simulink model "E_hyeok_RateError"  (R2023b)
settings: Solver=FixedStepAuto  StartTime=0.0  StopTime=inf  FixedStep=0.001  RelTol=1e-3  EnableMultiTasking=on
libraries: arduinolib x12, simulink x3, dspswit3 x2, spsOnDelayLib x2, arduinosensorlib x1
settings Model: ExtModeTrigDuration=2  Creator=user  LastModifiedBy=현대오토1
settings OptimizationCC: EnhancedBackFolding=on  PassReuseOutputArgsAs=Individual arguments  ZeroExternalMemoryAtStartup=off  ZeroInternalMemoryAtStartup=off  MaxStackSize=64  OptimizeBlockOrder=speed  DifferentSizesBufferReuse=on  OptimizationCustomize=off  EfficientTunableParamExpr=on
settings DebuggingCC: ParameterTunabilityLossMsg=error
settings HardwareCC: ProdBitPerInt=16  ProdBitPerPointer=16  ProdBitPerSizeT=16  ProdBitPerPtrDiffT=16  ProdLargestAtomicFloat=None  ProdWordSize=8  ProdHWDeviceType=Atmel->AVR
settings SFSimCC: MATLABDynamicMemAlloc=off
settings RTWCC: Description=Embedded Coder  SystemTargetFile=ert.tlc  HardwareBoard=Arduino Mega 2560  TemplateMakefile=ert_default_tmf  Toolchain=Arduino AVR  BuildConfiguration=Faster Runs
settings CodeAppCC: ForceParamTrailComments=on  IgnoreCustomStorageClasses=off  OperatorAnnotations=on  SimulinkDataObjDesc=on  SFDataObjDesc=on  InsertBlockDesc=on
settings ERTTargetCC: SupportContinuousTime=on  SupportVariableSizeSignals=on  ExtModeTransport=3  ExtModeStaticAlloc=on  ExtModeAutomaticAllocSize=off  ExtModeStaticAllocSize=2048  ExtModeMexFile=ext_xcp  ExtModeIntrfLevel=Level2 - Open

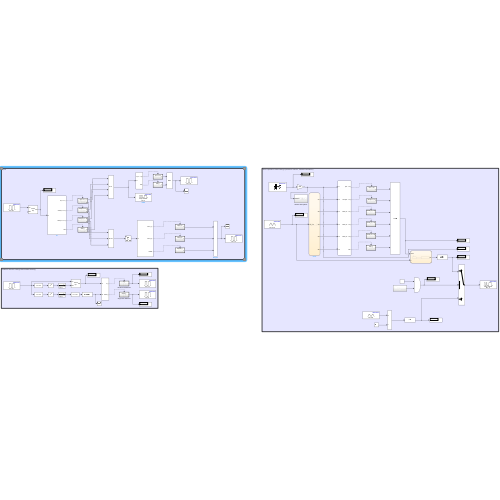
[thumbnail: Simulink's stored preview of the top-level diagram]
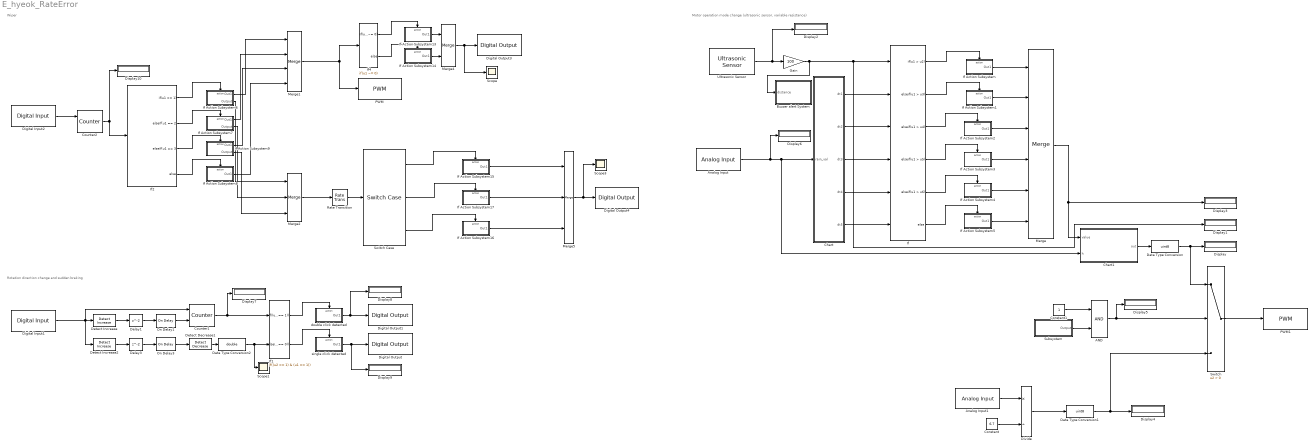
== system E_hyeok_RateError ==
  note: Wiper
  note: Motor operation mode change (ultrasonic sensor, variable resistance)
  note: Rotation direction change and sudden braking
  AND : Logic  IconShape=distinctive  AllPortsSameDT=off  OutDataTypeStr=boolean
  Analog Input : arduinolib/Analog Input  pinNumber=10  ReadResultsOnly=off  ConversionTriggerSource=Software  ExternalTriggerType=uint32( 0 )  OutputDataType=uint16  EnableConversionCompleteNotify=off  EnableOuputStatus=off  SampleTime=-1  blockPlatform=arduino
  Analog Input1 : arduinolib/Analog Input  pinNumber=8  ReadResultsOnly=off  ConversionTriggerSource=Software  ExternalTriggerType=uint32( 0 )  OutputDataType=uint16  EnableConversionCompleteNotify=off  EnableOuputStatus=off  SampleTime=-1  blockPlatform=arduino
  Buzzer alert System : Subsystem
  Chart : Stateflow chart  TreatAsAtomicUnit=on
  Chart1 : Stateflow chart  TreatAsAtomicUnit=on
      settings: PortSchema="{\"entries\":[{\"content\":{\"sides\":[{\"content\":{\"connectorIds\":[\"In2\",\"In1\"]},\"type\":\"ConnectorPlacement.EquallySpacedRectSide\",\"uuid\":\"b8bc21d1-4b9f-4189-a812-b41a4c5af9e6\"},{\"content\":{\"connectorIds\":[\"Out1\"],\"side\":\"RIGHT\"},\"type\":\"ConnectorPlacement.EquallySpacedRectSide\",\"uuid\":\"2c64dce3-08c2-4220-8c60-db9aba55cb61\"},{\"content\":{\"connectorIds\":[],\"side\":\"TOP\"},\"type\":\"ConnectorPlacement.EquallySpacedRectSide\",\"uuid\":\"e1e14768-a3b4-4969-ba09-2d2b4c878f0a\"}]},\"type\":\"ConnectorPlacement.EquallySpacedConnector\",\"uuid\":\"33700ad2-0727-43da-b85e-9713a6dc3065\"}],\"packageUris\":[\"http://schema.mathworks.com/mf0/Connector/R2020b\"],\"version\":\"1.0\"}"
  Constant : Constant  Value=6.7
  Constant1 : Constant
  Counter1 : dspswit3/Counter  Direction=Up  CountEvent=Rising edge  CounterSize=User defined  MaxCount=255  InitialCount=0  Output=Count  HitValue=32  ResetInput=on  SamplesPerFrame=1  Ts=1  CntDtype=double  HitDtype=Logical
  Counter2 : dspswit3/Counter  Direction=Up  CountEvent=Falling edge  CounterSize=User defined  MaxCount=3  InitialCount=0  Output=Count  HitValue=32  ResetInput=on  SamplesPerFrame=1  Ts=1  CntDtype=int8  HitDtype=Logical
  Data Type Conversion : DataTypeConversion  OutDataTypeStr=uint8  SaturateOnIntegerOverflow=off  RndMeth=Floor
  Data Type Conversion1 : DataTypeConversion  OutDataTypeStr=uint8  SaturateOnIntegerOverflow=off  RndMeth=Floor
  Data Type Conversion2 : DataTypeConversion  OutDataTypeStr=double  SaturateOnIntegerOverflow=off  RndMeth=Floor
  Delay1 : Delay
  Delay3 : Delay
  Detect Decrease1 : simulink/Logic and Bit Operations/Detect Decrease  vinit=0  OutDataTypeStr=uint8
  Detect Increase : simulink/Logic and Bit Operations/Detect Increase  vinit=1  OutDataTypeStr=boolean
  Detect Increase2 : simulink/Logic and Bit Operations/Detect Increase  vinit=1  OutDataTypeStr=boolean
  Digital Input1 : arduinolib/Digital Input  pinNumber=22  mode=Default  Direction=input  SampleTime=0.001  blockPlatform=arduino
  Digital Input2 : arduinolib/Digital Input  pinNumber=36  mode=Default  Direction=input  SampleTime=0.01  blockPlatform=arduino
  Digital Output : arduinolib/Digital Output  pinNumber=8  Direction=output  blockPlatform=arduino
  Digital Output1 : arduinolib/Digital Output  pinNumber=13  Direction=output  blockPlatform=arduino
  Digital Output3 : arduinolib/Digital Output  pinNumber=18  Direction=output  blockPlatform=arduino
  Digital Output4 : arduinolib/Digital Output  pinNumber=12  Direction=output  blockPlatform=arduino
  Display{,1..10} (11 alike) : Display
  Divide : Product  Inputs=*/
  Gain : Gain  Gain=100
  If : If  NumInputs=6  IfExpression=u1 > u2  ElseIfExpressions=u1 > u3, u1 > u4, u1 > u5, u1 > u6
  If Action Subsystem : Subsystem  TreatAsAtomicUnit=on
  If Action Subsystem1 : Subsystem  TreatAsAtomicUnit=on
  If Action Subsystem13 : Subsystem  TreatAsAtomicUnit=on
  If Action Subsystem14 : Subsystem  TreatAsAtomicUnit=on
  If Action Subsystem15 : Subsystem  TreatAsAtomicUnit=on
  If Action Subsystem16 : Subsystem  TreatAsAtomicUnit=on
  If Action Subsystem17 : Subsystem  TreatAsAtomicUnit=on
  If Action Subsystem2 : Subsystem  TreatAsAtomicUnit=on
  If Action Subsystem3 : Subsystem  TreatAsAtomicUnit=on
  If Action Subsystem4 : Subsystem  TreatAsAtomicUnit=on
  If Action Subsystem5 : Subsystem  TreatAsAtomicUnit=on
  If Action Subsystem6 : Subsystem  TreatAsAtomicUnit=on
  If Action Subsystem7 : Subsystem  TreatAsAtomicUnit=on
  If Action Subsystem8 : Subsystem  TreatAsAtomicUnit=on
  If Action Subsystem9 : Subsystem  TreatAsAtomicUnit=on
  If1 : If  NumInputs=2  IfExpression=(u2 == 1) & (u1 == 1)  ElseIfExpressions=(u2 == 1) & (u1 == 0)  ShowElse=off
  If2 : If  IfExpression=u1 == 1  ElseIfExpressions=u1 == 2, u1 == 3
  If4 : If  IfExpression=u1 ~= 0
  Merge : Merge  Inputs=6
  Merge1 : Merge  Inputs=4
  Merge2 : Merge  Inputs=3
  Merge4 : Merge
  Merge5 : Merge  Inputs=3
  On Delay1 : spsOnDelayLib/On Delay  DelayType=Off delay  delay=0.9  ic=0  Ts=0
  On Delay3 : spsOnDelayLib/On Delay  DelayType=Off delay  delay=0.9  ic=0  Ts=0
  PWM : arduinolib/PWM  pinNumber=3  frequencyType=Default  desiredFrequency=490.2  achievableFrequency=490.2
  PWM1 : arduinolib/PWM  pinNumber=11  frequencyType=Default  desiredFrequency=490.2  achievableFrequency=490.2
  Rate Transition : RateTransition  InitialCondition=0.01  OutPortSampleTime=0.001
  Scope : Scope
  Scope1 : Scope
  Scope3 : Scope
  Subsystem : Subsystem
  Switch : Switch  Criteria=u2 > Threshold  SaturateOnIntegerOverflow=off  InputSameDT=off
  Switch Case : SwitchCase  CaseConditions={1, 2}
  Ultrasonic Sensor : arduinosensorlib/Ultrasonic Sensor  NumSignalPins=2  TrigPin=50  EchoPin=51  SignalPin=3  SampleTime_=0.1  blockPlatform=ARDUINO
  double click detected : Subsystem  TreatAsAtomicUnit=on
  single click detected : Subsystem  TreatAsAtomicUnit=on
  wires:
  Ultrasonic Sensor/1 -> Gain/1, Display2/1
  Chart/1(dt1) -> If/2
  Chart/2(dt2) -> If/3
  Chart/3(dt3) -> If/4
  Chart/5(dt5) -> If/6
  Chart/4(dt4) -> If/5
  If Action Subsystem/1(Out1) -> Merge/1
  Gain/1 -> Buzzer alert System/1(distance), Display1/1, If/1
  If/2 -> If Action Subsystem1/Action
  If/3 -> If Action Subsystem2/Action
  If/4 -> If Action Subsystem3/Action
  If/5 -> If Action Subsystem4/Action
  If/6 -> If Action Subsystem5/Action
  If/1 -> If Action Subsystem/Action
  If Action Subsystem1/1(Out1) -> Merge/2
  If Action Subsystem2/1(Out1) -> Merge/3
  If Action Subsystem3/1(Out1) -> Merge/4
  If Action Subsystem4/1(Out1) -> Merge/5
  If Action Subsystem5/1(Out1) -> Merge/6
  Merge/1 -> Chart1/2(value), Display3/1
  Analog Input/1 -> Display6/1, Chart1/1(h), Chart/1(rain_val)
  Chart1/1(out) -> Data Type Conversion/1
  Data Type Conversion/1 -> Switch/1, Display/1
  AND/1 -> Display5/1, Switch/2
  Divide/1 -> Data Type Conversion1/1
  Switch/1 -> PWM1/1
  Constant1/1 -> AND/1
  Data Type Conversion1/1 -> Switch/3, Display4/1
  Constant/1 -> Divide/2
  Subsystem/1(Output) -> AND/2
  Analog Input1/1 -> Divide/1
  Detect Decrease1/1 -> Data Type Conversion2/1
  On Delay3/1 -> Detect Decrease1/1
  single click detected/1(Out1) -> Digital Output/1, Display9/1
  Detect Increase2/1 -> Delay3/1
  Delay3/1 -> On Delay3/1
  If1/2 -> single click detected/Action
  If1/1 -> double click detected/Action
  Counter1/1 -> Display7/1, If1/1
  Delay1/1 -> On Delay1/1
  Detect Increase/1 -> Delay1/1
  Data Type Conversion2/1 -> Scope1/1, If1/2
  Digital Input1/1 -> Counter1/1, Detect Increase2/1, Detect Increase/1
  double click detected/1(Out1) -> Digital Output1/1, Display8/1
  On Delay1/1 -> Counter1/2
  Merge4/1 -> Scope/1, Digital Output3/1
  If Action Subsystem7/2(Output) -> Merge2/2
  If Action Subsystem6/2(Output) -> Merge2/1
  If Action Subsystem14/1(Out1) -> Merge4/2
  If Action Subsystem13/1(Out1) -> Merge4/1
  Counter2/1 -> Display10/1, If2/1
  Merge1/1 -> If4/1, PWM/1
  If Action Subsystem9/2(Output) -> Merge2/3
  If2/4 -> If Action Subsystem8/Action
  Digital Input2/1 -> Counter2/1
  If2/1 -> If Action Subsystem6/Action
  If2/2 -> If Action Subsystem7/Action
  If2/3 -> If Action Subsystem9/Action
  If Action Subsystem6/1(Out1) -> Merge1/1
  If Action Subsystem7/1(Out1) -> Merge1/2
  If Action Subsystem9/1(Out1) -> Merge1/3
  If Action Subsystem8/1(Out1) -> Merge1/4
  If4/2 -> If Action Subsystem14/Action
  If4/1 -> If Action Subsystem13/Action
  Merge2/1 -> Rate Transition/1
  Merge5/1 -> Scope3/1, Digital Output4/1
  If Action Subsystem16/1(Out1) -> Merge5/3
  If Action Subsystem17/1(Out1) -> Merge5/2
  If Action Subsystem15/1(Out1) -> Merge5/1
  Switch Case/1 -> If Action Subsystem15/Action
  Switch Case/2 -> If Action Subsystem17/Action
  Switch Case/3 -> If Action Subsystem16/Action
  Rate Transition/1 -> Switch Case/1

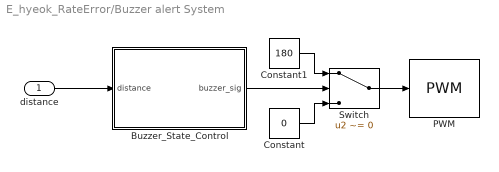
== system E_hyeok_RateError/Buzzer alert System ==
  distance : Inport
  Buzzer_State_Control : Stateflow chart  TreatAsAtomicUnit=on
  Constant : Constant  Value=0  OutDataTypeStr=uint8
  Constant1 : Constant  Value=180  OutDataTypeStr=uint8
  PWM : arduinolib/PWM  pinNumber=7  frequencyType=Specify  desiredFrequency=490.2  achievableFrequency=490.1961
  Switch : Switch  Criteria=u2 ~= 0  Threshold=1  SaturateOnIntegerOverflow=off  InputSameDT=off
  wires:
  Switch/1 -> PWM/1
  Constant/1 -> Switch/3
  Constant1/1 -> Switch/1
  Buzzer_State_Control/1(buzzer_sig) -> Switch/2
  distance/1 -> Buzzer_State_Control/1(distance)

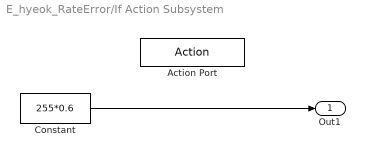
== system E_hyeok_RateError/If Action Subsystem ==
  Action Port : ActionPort  ActionPortLabel=if(u1 > u2)
  Constant : Constant  Value=255*0.6
  Out1 : Outport
  wires:
  Constant/1 -> Out1/1

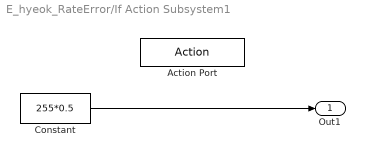
== system E_hyeok_RateError/If Action Subsystem1 ==
  Action Port : ActionPort  ActionPortLabel=elseif(u1 > u3)
  Constant : Constant  Value=255*0.5
  Out1 : Outport
  wires:
  Constant/1 -> Out1/1

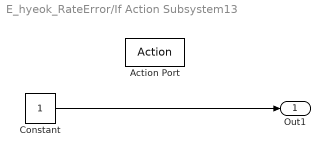
== system E_hyeok_RateError/If Action Subsystem13 ==
  Action Port : ActionPort  ActionPortLabel=if(u1 ~= 0)
  Constant : Constant
  Out1 : Outport
  wires:
  Constant/1 -> Out1/1

== system E_hyeok_RateError/If Action Subsystem14 ==
  Action Port : ActionPort  ActionPortLabel=else
  Constant : Constant  Value=0
  Out1 : Outport
  wires:
  Constant/1 -> Out1/1

== system E_hyeok_RateError/If Action Subsystem15 ==
  Action Port : ActionPort  ActionPortLabel=case [ 1 ]:
  Pulse Generator : DiscretePulseGenerator  PulseType=Time based  PulseWidth=50  PhaseDelay=0.01
  Out1 : Outport
  wires:
  Pulse Generator/1 -> Out1/1

== system E_hyeok_RateError/If Action Subsystem16 ==
  Action Port : ActionPort  ActionPortLabel=default:
  Pulse Generator : DiscretePulseGenerator  PulseType=Time based  Period=6  PulseWidth=50  PhaseDelay=0.01
  Out1 : Outport
  wires:
  Pulse Generator/1 -> Out1/1

== system E_hyeok_RateError/If Action Subsystem17 ==
  Action Port : ActionPort  ActionPortLabel=case [ 2 ]:
  Pulse Generator : DiscretePulseGenerator  PulseType=Time based  Period=4  PulseWidth=50  PhaseDelay=0.01  VectorParams1D=off
  Out1 : Outport
  wires:
  Pulse Generator/1 -> Out1/1

== system E_hyeok_RateError/If Action Subsystem2 ==
  Action Port : ActionPort  ActionPortLabel=elseif( u1 > u4)
  Constant : Constant  Value=255*0.4
  Out1 : Outport
  wires:
  Constant/1 -> Out1/1

== system E_hyeok_RateError/If Action Subsystem3 ==
  Action Port : ActionPort  ActionPortLabel=elseif( u1 > u5)
  Constant : Constant  Value=255*0.3
  Out1 : Outport
  wires:
  Constant/1 -> Out1/1

== system E_hyeok_RateError/If Action Subsystem4 ==
  Action Port : ActionPort  ActionPortLabel=elseif( u1 > u6)
  Constant : Constant  Value=255*0.2
  Out1 : Outport
  wires:
  Constant/1 -> Out1/1

== system E_hyeok_RateError/If Action Subsystem5 ==
  Action Port : ActionPort  ActionPortLabel=else
  Constant : Constant  Value=255*0
  Out1 : Outport
  wires:
  Constant/1 -> Out1/1

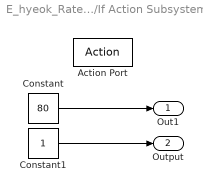
== system E_hyeok_RateError/If Action Subsystem6 ==
  Action Port : ActionPort  ActionPortLabel=if(u1 == 1)
  Constant : Constant  Value=80
  Constant1 : Constant
  Out1 : Outport
  Output : Outport  Port=2
  wires:
  Constant/1 -> Out1/1
  Constant1/1 -> Output/1

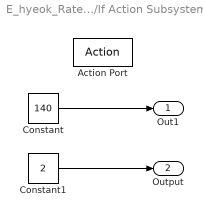
== system E_hyeok_RateError/If Action Subsystem7 ==
  Action Port : ActionPort  ActionPortLabel=elseif(u1 == 2)
  Constant : Constant  Value=140
  Constant1 : Constant  Value=2
  Out1 : Outport
  Output : Outport  Port=2
  wires:
  Constant/1 -> Out1/1
  Constant1/1 -> Output/1

== system E_hyeok_RateError/If Action Subsystem8 ==
  Action Port : ActionPort  ActionPortLabel=else
  Constant : Constant  Value=0
  Out1 : Outport
  wires:
  Constant/1 -> Out1/1

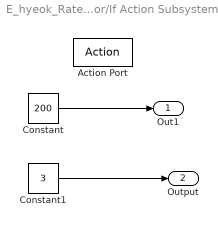
== system E_hyeok_RateError/If Action Subsystem9 ==
  Action Port : ActionPort  ActionPortLabel=elseif( u1 == 3)
  Constant : Constant  Value=200
  Constant1 : Constant  Value=3
  Out1 : Outport
  Output : Outport  Port=2
  wires:
  Constant/1 -> Out1/1
  Constant1/1 -> Output/1

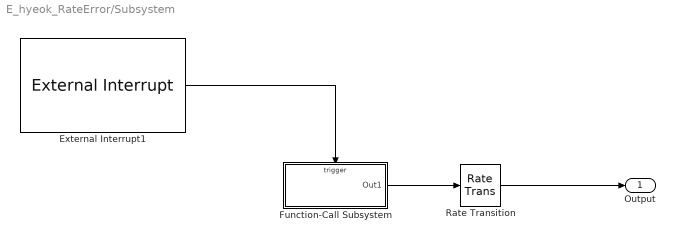
== system E_hyeok_RateError/Subsystem ==
  External Interrupt1 : arduinolib/External Interrupt  Pin=2  PullUp=off  Mode=FALLING  InterruptSimulationInput=off
  Function-Call Subsystem : Subsystem  TreatAsAtomicUnit=on
  Rate Transition : RateTransition  Deterministic=off
  Output : Outport
  wires:
  Function-Call Subsystem/1(Out1) -> Rate Transition/1
  External Interrupt1/1 -> Function-Call Subsystem/Trigger
  Rate Transition/1 -> Output/1

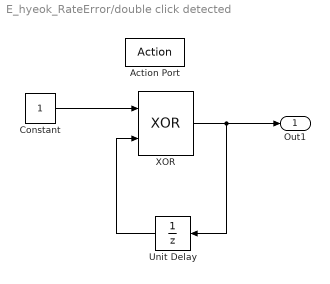
== system E_hyeok_RateError/double click detected ==
  Action Port : ActionPort  ActionPortLabel=if((u2 == 1) & (u1 == 1))
  Constant : Constant
  Unit Delay : UnitDelay  SampleTime=-1  HasFrameUpgradeWarning=on
  XOR : Logic  Operator=XOR  IconShape=distinctive  AllPortsSameDT=off  OutDataTypeStr=boolean
  Out1 : Outport
  wires:
  Constant/1 -> XOR/1
  XOR/1 -> Unit Delay/1, Out1/1
  Unit Delay/1 -> XOR/2

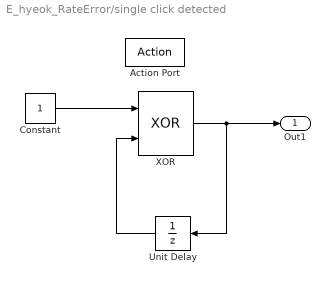
== system E_hyeok_RateError/single click detected ==
  Action Port : ActionPort  ActionPortLabel=elseif((u2 == 1) & (u1 == 0))
  Constant : Constant
  Unit Delay : UnitDelay  SampleTime=-1  HasFrameUpgradeWarning=on
  XOR : Logic  Operator=XOR  IconShape=distinctive  AllPortsSameDT=off  OutDataTypeStr=boolean
  Out1 : Outport
  wires:
  Unit Delay/1 -> XOR/2
  XOR/1 -> Out1/1, Unit Delay/1
  Constant/1 -> XOR/1

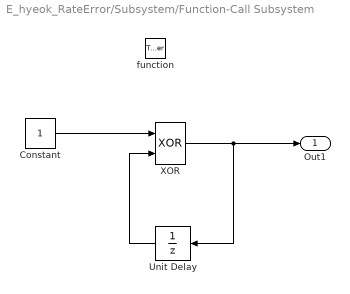
== system E_hyeok_RateError/Subsystem/Function-Call Subsystem ==
  function : TriggerPort  TriggerType=function-call  VariantControl=(inherit)
  Constant : Constant
  Unit Delay : UnitDelay  InitialCondition=1  SampleTime=-1  HasFrameUpgradeWarning=on
  XOR : Logic  Operator=XOR  IconShape=distinctive  AllPortsSameDT=off  OutDataTypeStr=boolean
  Out1 : Outport
  wires:
  Constant/1 -> XOR/1
  XOR/1 -> Unit Delay/1, Out1/1
  Unit Delay/1 -> XOR/2

== stateflow chart E_hyeok_RateError/Chart1 ==
  state not_rain
    out = value
  state rain
    out = value - (((255*0.6) - value) *0.5)
  (default) -> not_rain
  not_rain -> rain : [h<=800]
  rain -> not_rain : [h>800]
  data: h input; value input; out output

== stateflow chart E_hyeok_RateError/Buzzer alert System/Buzzer_State_Control ==
  state Buzzer_Mode1
    state p1
      period = 0.7;
      state bz_on2
        buzzer_sig = 1;
      state bz_off1
        buzzer_sig = 0;
      state bz_start
      Buzzer_Mode1.p1.bz_off1 -> Buzzer_Mode1.p1.bz_on2 : after(period,sec)
      Buzzer_Mode1.p1.bz_on2 -> Buzzer_Mode1.p1.bz_off1 : after(period,sec)
      Buzzer_Mode1.p1.bz_start -> Buzzer_Mode1.p1.bz_on2 [order 1] : [buzzer_sig==0]
      Buzzer_Mode1.p1.bz_start -> Buzzer_Mode1.p1.bz_off1 [order 2] : [buzzer_sig==1]
      (default) -> Buzzer_Mode1.p1.bz_start
    state p2
      period = 0.5;
      state bz_on2
        buzzer_sig = 1;
      state bz_off1
        buzzer_sig = 0;
      state bz_start
      Buzzer_Mode1.p2.bz_off1 -> Buzzer_Mode1.p2.bz_on2 : after(period,sec)
      Buzzer_Mode1.p2.bz_on2 -> Buzzer_Mode1.p2.bz_off1 : after(period,sec)
      Buzzer_Mode1.p2.bz_start -> Buzzer_Mode1.p2.bz_on2 [order 1] : [buzzer_sig==0]
      Buzzer_Mode1.p2.bz_start -> Buzzer_Mode1.p2.bz_off1 [order 2] : [buzzer_sig==1]
      (default) -> Buzzer_Mode1.p2.bz_start
    state p4
      period = 0.1;
      state bz_on2
        buzzer_sig = 1;
      state bz_off1
        buzzer_sig = 0;
      state bz_start
      Buzzer_Mode1.p4.bz_off1 -> Buzzer_Mode1.p4.bz_on2 : after(period,sec)
      Buzzer_Mode1.p4.bz_on2 -> Buzzer_Mode1.p4.bz_off1 : after(period,sec)
      Buzzer_Mode1.p4.bz_start -> Buzzer_Mode1.p4.bz_on2 [order 1] : [buzzer_sig==0]
      Buzzer_Mode1.p4.bz_start -> Buzzer_Mode1.p4.bz_off1 [order 2] : [buzzer_sig==1]
      (default) -> Buzzer_Mode1.p4.bz_start
    state p3
      period = 0.3;
      state bz_on2
        buzzer_sig = 1;
      state bz_off1
        buzzer_sig = 0;
      state bz_start
      Buzzer_Mode1.p3.bz_off1 -> Buzzer_Mode1.p3.bz_on2 : after(period,sec)
      Buzzer_Mode1.p3.bz_on2 -> Buzzer_Mode1.p3.bz_off1 : after(period,sec)
      Buzzer_Mode1.p3.bz_start -> Buzzer_Mode1.p3.bz_on2 [order 1] : [buzzer_sig==0]
      Buzzer_Mode1.p3.bz_start -> Buzzer_Mode1.p3.bz_off1 [order 2] : [buzzer_sig==1]
      (default) -> Buzzer_Mode1.p3.bz_start
    (default) -> p1
    p2 -> p1 [order 1] : [distance>40]
    p1 -> p2 [order 1] : [distance>30&distance<=40]
    p4 -> p1 [order 1] : [distance>40]
    p1 -> p4 [order 2] : [distance>10&distance<=20]
    p3 -> p1 [order 1] : [distance>40]
    p1 -> p3 [order 3] : [distance>20&distance<=30]
    p3 -> p2 [order 2] : [distance>30&distance<=40]
    p2 -> p3 [order 3] : [distance>20&distance<=30]
    p2 -> p4 [order 2] : [distance>10&distance<=20]
    p4 -> p2 [order 2] : [distance>30&distance<=40]
    p3 -> p4 [order 3] : [distance>10&distance<=20]
    p4 -> p3 [order 3] : [distance>20&distance<=30]
  state Buzzer_Standby
    buzzer_sig = 0;
  state Buzzer_Mode2
    buzzer_sig = 1;
  state bz_on [commented out]
    buzzer_sig = 1;
  state bz_off [commented out]
    buzzer_sig = 0;
  state bz_start [commented out]
  (default) -> Buzzer_Standby
  Buzzer_Standby -> Buzzer_Mode1 [order 1] : [distance<=50]
  Buzzer_Mode1 -> Buzzer_Standby [order 2] : [distance>50]
  Buzzer_Mode2 -> Buzzer_Standby [order 2] : [distance>50]
  Buzzer_Standby -> Buzzer_Mode2 [order 2] : [distance<=10]
  Buzzer_Mode2 -> Buzzer_Mode1 [order 1] : [distance>10]
  Buzzer_Mode1 -> Buzzer_Mode2 [order 1] : [distance<=10]
  bz_off -> bz_on [commented out] : after(period,sec)
  bz_on -> bz_off [commented out] : after(period,sec)
  bz_start -> bz_on [commented out] : [buzzer_sig==1]
  bz_start -> bz_off [commented out] : [buzzer_sig==0]
  (default) -> bz_start [commented out]
  data: distance input; buzzer_sig output; period local

== stateflow chart E_hyeok_RateError/Chart ==
  state Non_rain
    dt1 = 25
    dt2 = 20
    dt3 = 15
    dt4 = 10
    dt5 = 5
  state Rain
    dt1=35
    dt2=30
    dt3=25
    dt4=20
    dt5=15
  (default) -> Non_rain
  Rain -> Non_rain : [rain_val > 800]
  Non_rain -> Rain : [rain_val <= 800]
  data: dt1 output; dt2 output; dt3 output; dt4 output; dt5 output; rain_val input
